simulink model "simulink_s1_22b"  (R2023b)
settings: Solver=VariableStepAuto  StartTime=0.0  StopTime=15  RelTol=1e-3
values from neighbouring files (symbols this model uses):
  OUT = [0 0.001 0.002 0.003 0.004 0.005 0.006 0.007 0.008 0.009 0.01 0.011 ... (30000 elements, 15000x2)]    [kp=4.2-data.mat]    (also in kp=8.7-data.mat; script_s1.m = [time, data(:,1)])
settings Model: Creator=Admin  LastModifiedBy=lucasp
settings SolverCC: AlgebraicLoopSolver=TrustRegion

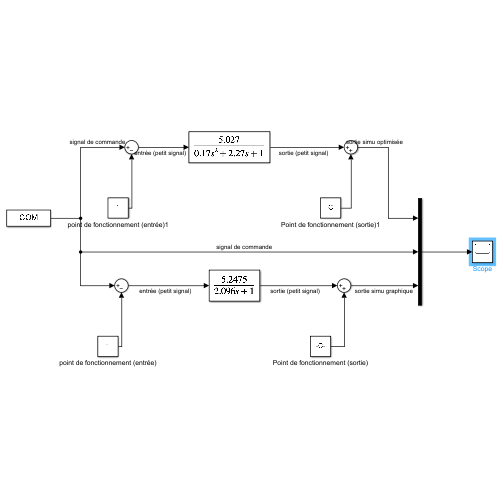
[thumbnail: Simulink's stored preview of the top-level diagram]
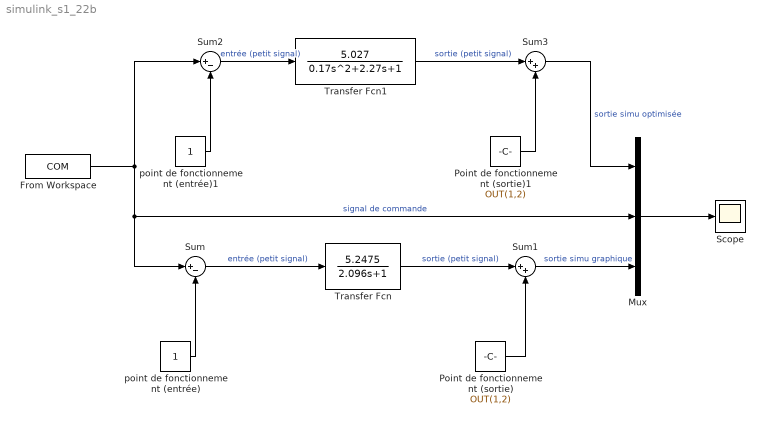
== system simulink_s1_22b ==
  From Workspace : FromWorkspace  VariableName=COM
  Mux : Mux  Inputs=3
  Point de fonctionnement (sortie) : Constant  Value=OUT(1,2)
  Point de fonctionnement (sortie)1 : Constant  Value=OUT(1,2)
  Scope : Scope
  Sum : Sum  Inputs=|+-
  Sum1 : Sum  Inputs=|++
  Sum2 : Sum  Inputs=|+-
  Sum3 : Sum  Inputs=|++
  Transfer Fcn : TransferFcn  Numerator=[5.2475]  Denominator=[2.096 1]
  Transfer Fcn1 : TransferFcn  Numerator=[5.027]  Denominator=[0.17 2.27 1]
  point de fonctionnement (entrée) : Constant
  point de fonctionnement (entrée)1 : Constant
  wires:
  Sum/1 -> Transfer Fcn/1  "entrée (petit signal)"
  Sum3/1 -> Mux/1  "sortie simu optimisée"
  Transfer Fcn/1 -> Sum1/1  "sortie (petit signal)"
  Mux/1 -> Scope/1
  Point de fonctionnement (sortie)/1 -> Sum1/2
  point de fonctionnement (entrée)/1 -> Sum/2
  Sum1/1 -> Mux/3  "sortie simu graphique"
  Sum2/1 -> Transfer Fcn1/1  "entrée (petit signal)"
  From Workspace/1 -> Sum2/1, Sum/1, Mux/2  "signal de commande"
  point de fonctionnement (entrée)1/1 -> Sum2/2
  Transfer Fcn1/1 -> Sum3/1  "sortie (petit signal)"
  Point de fonctionnement (sortie)1/1 -> Sum3/2
